simulink model "velo_model"  (R2022a)
settings: Solver=ode1  StartTime=0.0  StopTime=Ts  FixedStep=0.01  RelTol=1e-3
values from neighbouring files (symbols this model uses):
  L = 3    [MultiAgent_initiateSAC.m]    (also in control_velocity.m; initiate.m; initiateHybrid.m; initiateSAC.m)
  ld = 5    [MultiAgent_initiateSAC.m]    (also in control_velocity.m; initiate.m; initiateHybrid.m; initiateSAC.m)
  psi_o = 0    [MultiAgent_initiateSAC.m]    (also in control_velocity.m; initiate.m; initiateHybrid.m = thetaRefs(1)*(pi/180); initiateSAC.m)
  Ts = 100    [MultiAgent_initiateSAC.m]    (also in control_velocity.m; initiate.m; initiateHybrid.m = 50; initiateSAC.m)
  vel = 5    [MultiAgent_initiateSAC.m]    (also in control_velocity.m = 7; initiate.m = 10; initiateHybrid.m; initiateSAC.m)
  X_o = refPose(1,1)+0    [MultiAgent_initiateSAC.m]    (also in control_velocity.m; initiate.m = refPose(1,1)+60; initiateHybrid.m = xRef(1); initiateSAC.m)
  xRef = refPose(:,1)    [MultiAgent_initiateSAC.m]    (also in control_velocity.m; initiate.m; initiateHybrid.m; initiateSAC.m)
  Y_o = -refPose(1,2)+20    [MultiAgent_initiateSAC.m]    (also in control_velocity.m = -refPose(1,2)+0; initiate.m; initiateHybrid.m = yRef(1); initiateSAC.m = -refPose(1,2)+0)
  yRef = -refPose(:,2)    [MultiAgent_initiateSAC.m]    (also in control_velocity.m; initiate.m; initiateHybrid.m; initiateSAC.m)
libraries: vehdynlibviscommon x1, robotalgslib x1, rllib x1, autolibshared x1
settings Model: Creator=berka  LastModifiedBy=berka
settings DebuggingCC: UnconnectedInputMsg=warning  UnconnectedOutputMsg=warning  UnconnectedLineMsg=warning
settings RTWCC: DLArmComputeVersion=19.05

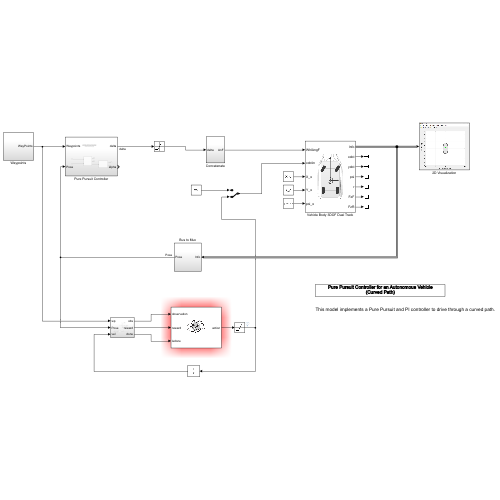
[thumbnail: Simulink's stored preview of the top-level diagram]
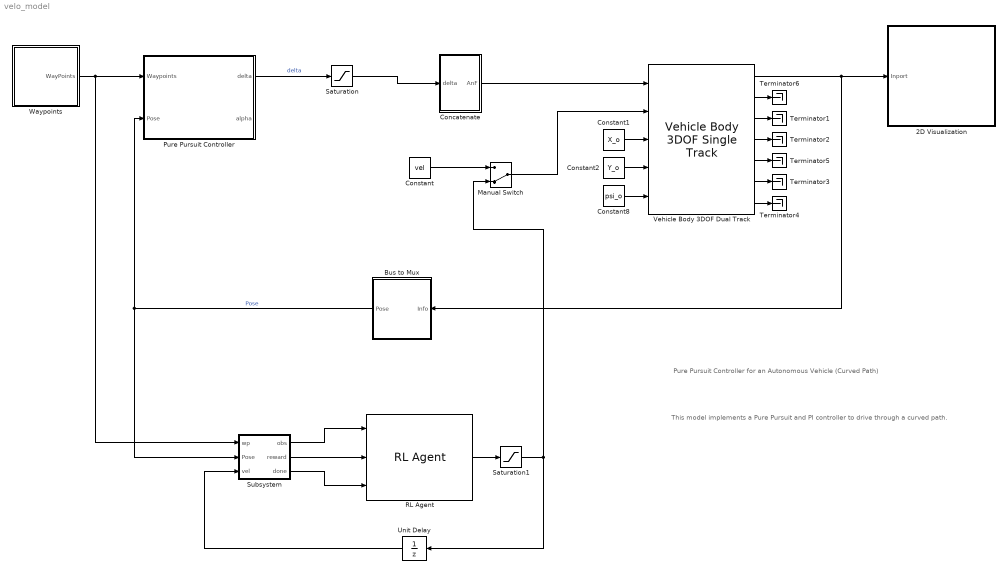
== system velo_model ==
  note: This model implements a Pure Pursuit and PI controller to drive through a curved path.
  note: Pure Pursuit Controller for an Autonomous Vehicle
      | (Curved Path)
  2D Visualization : Subsystem
      mask Display: image("visualization.JPG");
  Bus to Mux : Subsystem
  Concatenate : Subsystem
  Constant : Constant  Value=vel
  Constant1 : Constant  Value=X_o
  Constant2 : Constant  Value=Y_o
  Constant8 : Constant  Value=psi_o
  Manual Switch : ManualSwitch  CurrentSetting=0
  Pure Pursuit Controller : Subsystem
  RL Agent : rllib/RL Agent  Agent=agent  ExternalActionAsInput=off  ProvideLastAction=off  ProvideCumRwd=off  TreatAsDirectFeedthrough=on  UseStrictObservationDataTypes=off
  Saturation : Saturate
  Saturation1 : Saturate  UpperLimit=15  LowerLimit=1
  Subsystem : Subsystem
  Terminator{1..6} (6 alike) : Terminator
  Unit Delay : UnitDelay  SampleTime=-1  HasFrameUpgradeWarning=on
  Vehicle Body 3DOF Dual Track : autolibshared/Vehicle Body 3DOF Single Track  trackMode=Dual  inputMode=External longitudinal velocity  frontSteerMode=on  rearSteerMode=off  windMode=off  muMode=off  extFMode=off  extMMode=off  htchFMode=off  htchMMode=off  extXo=on  extpsio=on  extxdoto=off  extro=off  extYo=on  extTamb=off  extydoto=off  aMode=2  NF=2  NR=2  m=2000  a=1.4  b=1.6  h=0.35  dh=1  hh=0.2  X_o=0  xdot_o=0  CalphaMode=off  sigmaMode=on  d=0  hl=0  w=[1.4,1.4]  Cy_f=12e3  Cy_r=11e3  sigma_f=.1  sigma_r=.1  alpha_f_brk=[-.1 .1]  Cy_f_data=[-9e3 9e3]  alpha_r_brk=[-.1 .1]  Cy_r_data=[-9e3 9e3]  Y_o=0  ydot_o=0  Izz=4000  psi_o=0  r_o=0  Af=2  Cd=.3  Cl=.1  Cpm=.1  beta_w=[0:0.01:0.3]  Cs=[0:0.03:0.9]  Cym=[0:0.01:0.3]  Pabs=101325  Tair=273  g=9.81  mu=1  xdot_tol=.01  Fznom=5000  Fxtire_sat=7e4  Fytire_sat=7e4  longOff=0  latOff=0  vertOff=0  wrapAng=off
      settings: SourceProductBaseCode=PW,DR,MT,VE
  Waypoints : Subsystem
  wires:
  Vehicle Body 3DOF Dual Track/2 -> Terminator6/1
  Constant1/1 -> Vehicle Body 3DOF Dual Track/3
  Vehicle Body 3DOF Dual Track/3 -> Terminator1/1
  Vehicle Body 3DOF Dual Track/1 -> 2D Visualization/1(Inport), Bus to Mux/1(Info)
  Constant8/1 -> Vehicle Body 3DOF Dual Track/5
  Concatenate/1(AnF) -> Vehicle Body 3DOF Dual Track/1
  Vehicle Body 3DOF Dual Track/6 -> Terminator3/1
  Constant2/1 -> Vehicle Body 3DOF Dual Track/4
  Vehicle Body 3DOF Dual Track/7 -> Terminator4/1
  Vehicle Body 3DOF Dual Track/4 -> Terminator2/1
  Vehicle Body 3DOF Dual Track/5 -> Terminator5/1
  Waypoints/1(WayPoints) -> Subsystem/1(wp), Pure Pursuit Controller/1(Waypoints)
  Bus to Mux/1(Pose) -> Subsystem/2(Pose), Pure Pursuit Controller/2(Pose)  "Pose"
  Saturation/1 -> Concatenate/1(delta)
  Pure Pursuit Controller/1(delta) -> Saturation/1  "delta"
  Subsystem/1(obs) -> RL Agent/1
  Subsystem/2(reward) -> RL Agent/2
  Subsystem/3(done) -> RL Agent/3
  RL Agent/1 -> Saturation1/1
  Saturation1/1 -> Unit Delay/1, Manual Switch/2
  Unit Delay/1 -> Subsystem/3(vel)
  Manual Switch/1 -> Vehicle Body 3DOF Dual Track/2
  Constant/1 -> Manual Switch/1

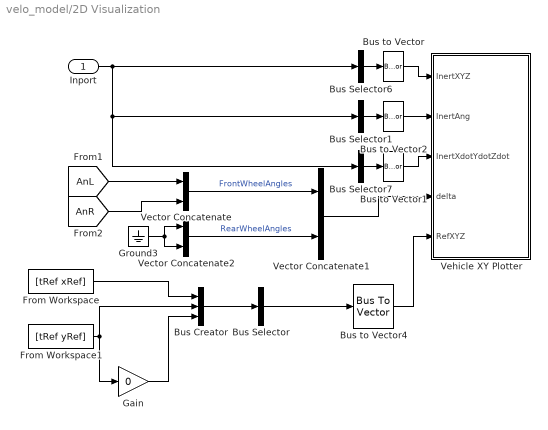
== system velo_model/2D Visualization ==
  Inport : Inport
  Bus Creator : BusCreator  Inputs=3
  Bus Selector : BusSelector  OutputSignals=signal1,signal2,signal3  OutputAsBus=on
  Bus Selector1 : BusSelector  OutputSignals=InertFrm.Cg.Ang.phi,InertFrm.Cg.Ang.theta,InertFrm.Cg.Ang.psi  OutputAsBus=on
  Bus Selector6 : BusSelector  OutputSignals=InertFrm.Geom.Disp.X,InertFrm.Geom.Disp.Y,InertFrm.Geom.Disp.Z  OutputAsBus=on
  Bus Selector7 : BusSelector  OutputSignals=InertFrm.Geom.Vel.Xdot,InertFrm.Geom.Vel.Ydot,InertFrm.Geom.Vel.Zdot  OutputAsBus=on
  Bus to Vector{,1..2,4} (4 alike) : BusToVector
  From Workspace : FromWorkspace  VariableName=[tRef xRef]
  From Workspace1 : FromWorkspace  VariableName=[tRef yRef]
  Gain : Gain  Gain=0
  Ground3 : Ground
  Vector Concatenate : Concatenate
  Vector Concatenate1 : Concatenate
  Vector Concatenate2 : Concatenate
  Vehicle XY Plotter : Subsystem  mask(Vehicle XY Plotter){a=2, b=2, w=2, figBorder=10, bufferSize=1024, extRef=on, pltDT=.2}
      mask prompts: a "Distance to front axle from CG, a [m]:"; b "Distance to rear axle from CG, b [m]:"; w "Track width, w [m]:"; figBorder "Distance to figure borders, figBorder [m]:"; bufferSize "Path buffer sampe size, bufferSize []:"; extRef "Plot path reference, extRef"; pltDT "Plot update rate, pltDT [s]:"
      mask help:
      | This block will display a MATLAB figure which indicates the vehicle path, current position and heading velocity.
      | An optional path reference is also provided.
      mask init:
      | if autoblkschecksimstopped(gcb)
      |     PortName = 'RefXYZ';
      |     InportOption  = {'built-in/Ground', [PortName, ' Ground'];...
      |         'built-in/Inport',PortName };
      |     if ~strcmp(get_param(gcb,'extRef'),'on')
      |         NewBlkHdl = autoblksreplaceblock(gcb, InportOption, 1);
      |         set_param(NewBlkHdl, 'ShowName', 'off');
      |     else
      |         autoblksreplaceblock(gcb, InportOption, 2);
      |     end
      | end
      mask TypeOptions a: Vehicle XY Plotter/a
      mask TypeOptions b: Vehicle XY Plotter/b
      mask TypeOptions w: Vehicle XY Plotter/w
      mask TypeOptions figBorder: Vehicle XY Plotter/figBorder
      mask TypeOptions bufferSize: Vehicle XY Plotter/bufferSize
  wires:
  Vector Concatenate1/1 -> Vehicle XY Plotter/4(delta)
  Ground3/1 -> Vector Concatenate2/1, Vector Concatenate2/2
  Bus Selector6/1 -> Bus to Vector/1
  Vector Concatenate/1 -> Vector Concatenate1/1  "FrontWheelAngles"
  [AnL] -> Vector Concatenate/1
  Vector Concatenate2/1 -> Vector Concatenate1/2  "RearWheelAngles"
  Bus Selector7/1 -> Bus to Vector1/1
  Bus to Vector1/1 -> Vehicle XY Plotter/3(InertXdotYdotZdot)
  Bus to Vector/1 -> Vehicle XY Plotter/1(InertXYZ)
  Bus to Vector2/1 -> Vehicle XY Plotter/2(InertAng)
  Bus Selector1/1 -> Bus to Vector2/1
  [AnR] -> Vector Concatenate/2
  Inport/1 -> Bus Selector7/1, Bus Selector1/1, Bus Selector6/1
  Bus to Vector4/1 -> Vehicle XY Plotter/5(RefXYZ)
  Bus Selector/1 -> Bus to Vector4/1
  From Workspace1/1 -> Gain/1, Bus Creator/2
  Gain/1 -> Bus Creator/3
  From Workspace/1 -> Bus Creator/1
  Bus Creator/1 -> Bus Selector/1

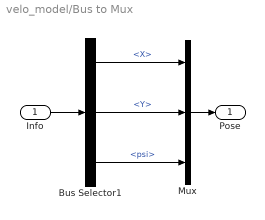
== system velo_model/Bus to Mux ==
  Info : Inport
  Bus Selector1 : BusSelector  OutputSignals=InertFrm.Cg.Disp.X,InertFrm.Cg.Disp.Y,InertFrm.Cg.Ang.psi
  Mux : Mux  Inputs=3
  Pose : Outport
  wires:
  Bus Selector1/3 -> Mux/3  "<psi>"
  Bus Selector1/1 -> Mux/1  "<X>"
  Mux/1 -> Pose/1
  Bus Selector1/2 -> Mux/2  "<Y>"
  Info/1 -> Bus Selector1/1

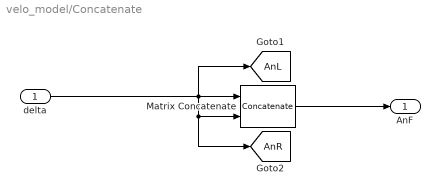
== system velo_model/Concatenate ==
  delta : Inport
  Matrix Concatenate : Concatenate
  AnF : Outport  VectorParamsAs1DForOutWhenUnconnected=off
  tag scope: AnL=global, AnR=global
  wires:
  Matrix Concatenate/1 -> AnF/1
  delta/1 -> [AnL], [AnR], Matrix Concatenate/2, Matrix Concatenate/1

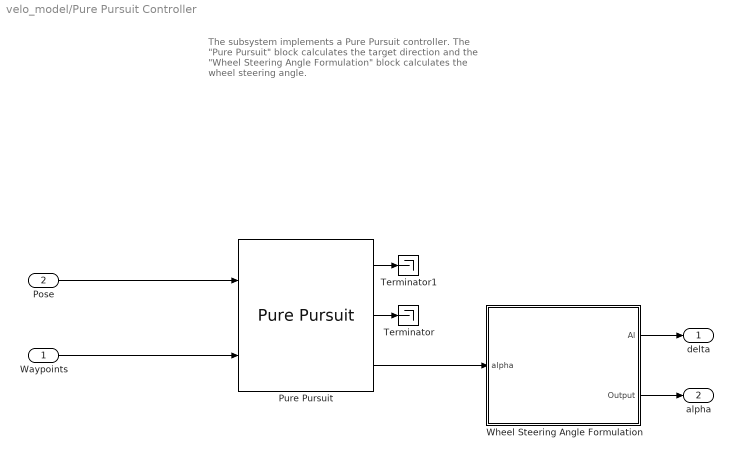
== system velo_model/Pure Pursuit Controller ==
  note: The subsystem implements a Pure Pursuit controller. The "Pure Pursuit" block calculates the target direction and the "Wheel Steering Angle Formulation" block calculates the wheel steering angle.
  Waypoints : Inport
  Pose : Inport  Port=2
  Pure Pursuit : robotalgslib/Pure Pursuit  DesiredLinearVelocity=vel  MaxAngularVelocity=1.0  LookaheadDistance=2.2754  TargetDirPort=on  SimulateUsing=Code generation
  Terminator : Terminator
  Terminator1 : Terminator
  Wheel Steering Angle Formulation : Subsystem  mask{L=L, ld=ld}
      mask prompts: L "Bicycle length"; ld "Lookahead distance"
      mask TypeOptions L: Bicycle length/Value
      mask TypeOptions ld: Lookahead distance/Value
      mask Display:
      | image("GeometryMask.png")
      | port_label('input', 1, 'alpha')
      | port_label('output', 1, 'delta')
  delta : Outport
  alpha : Outport  Port=2
  wires:
  Pure Pursuit/3 -> Wheel Steering Angle Formulation/1(alpha)
  Waypoints/1 -> Pure Pursuit/2
  Pose/1 -> Pure Pursuit/1
  Pure Pursuit/1 -> Terminator1/1
  Pure Pursuit/2 -> Terminator/1
  Wheel Steering Angle Formulation/1(Al) -> delta/1
  Wheel Steering Angle Formulation/2(Output) -> alpha/1

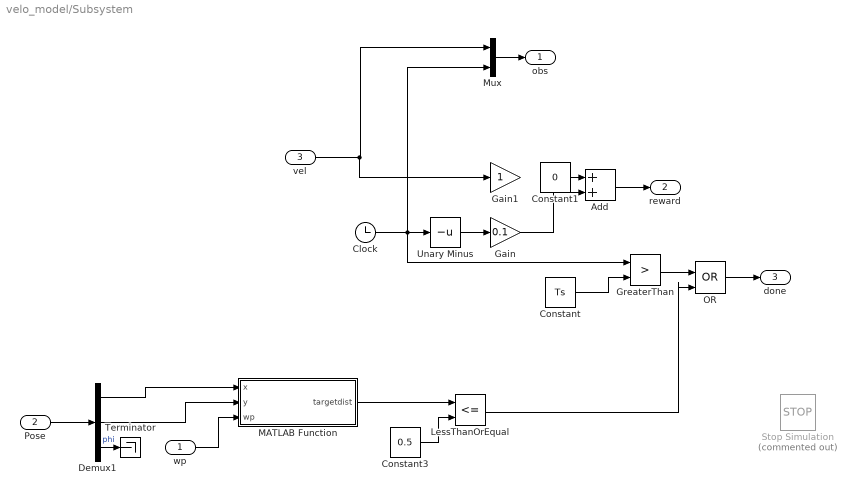
== system velo_model/Subsystem ==
  wp : Inport
  Pose : Inport  Port=2
  vel : Inport  Port=3
  Add : Sum
  Clock : Clock
  Constant : Constant  Value=Ts
  Constant1 : Constant  Value=0
  Constant3 : Constant  Value=0.5
  Demux1 : Demux  Outputs=3
  Gain : Gain  Gain=0.1
  Gain1 : Gain
  GreaterThan : RelationalOperator  Operator=>  OutDataTypeStr=boolean  RndMeth=Simplest  InputSameDT=off
  LessThanOrEqual : RelationalOperator  Operator=<=  OutDataTypeStr=boolean  RndMeth=Simplest  InputSameDT=off
  MATLAB Function : MATLAB Function  TreatAsAtomicUnit=on
  Mux : Mux  Inputs=2
  OR : Logic  Operator=OR  IconShape=distinctive  AllPortsSameDT=off  OutDataTypeStr=boolean
  Stop Simulation : Stop  Commented=on
  Terminator : Terminator
  Unary Minus : UnaryMinus
  obs : Outport
  reward : Outport  Port=2
  done : Outport  Port=3
  wires:
  Demux1/3 -> Terminator/1  "phi"
  Constant3/1 -> LessThanOrEqual/2
  Clock/1 -> GreaterThan/1, Mux/2, Unary Minus/1
  Pose/1 -> Demux1/1
  Unary Minus/1 -> Gain/1
  Demux1/1 -> MATLAB Function/1(x)
  MATLAB Function/1(targetdist) -> LessThanOrEqual/1
  Demux1/2 -> MATLAB Function/2(y)
  wp/1 -> MATLAB Function/3(wp)
  vel/1 -> Gain1/1, Mux/1
  Mux/1 -> obs/1
  Add/1 -> reward/1
  Gain/1 -> Add/2
  Constant/1 -> GreaterThan/2
  GreaterThan/1 -> OR/1
  LessThanOrEqual/1 -> OR/2
  OR/1 -> done/1
  Constant1/1 -> Add/1

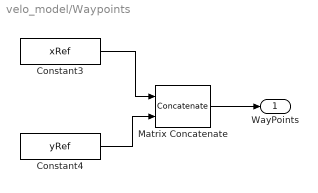
== system velo_model/Waypoints ==
  Constant3 : Constant  Value=xRef  SampleTime=0.1
  Constant4 : Constant  Value=yRef  SampleTime=0.1
  Matrix Concatenate : Concatenate  Mode=Multidimensional array  ConcatenateDimension=2
  WayPoints : Outport
  wires:
  Constant4/1 -> Matrix Concatenate/2
  Matrix Concatenate/1 -> WayPoints/1
  Constant3/1 -> Matrix Concatenate/1

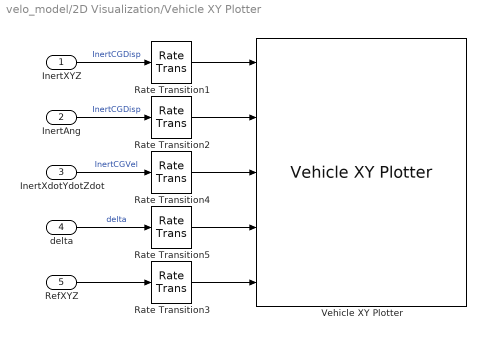
== system velo_model/2D Visualization/Vehicle XY Plotter ==
  InertXYZ : Inport
  InertAng : Inport  Port=2
  InertXdotYdotZdot : Inport  Port=3
  delta : Inport  Port=4
  RefXYZ : Inport  Port=5
  Rate Transition{1..5} (5 alike) : RateTransition  Deterministic=off  OutPortSampleTime=pltDT
  Vehicle XY Plotter : vehdynlibviscommon/Vehicle XY Plotter  w=w  a=a  b=b  figBorder=figBorder  bufferSize=bufferSize  extStats=off  extTireF=off
      settings: SourceProductBaseCode=VE
  wires:
  Rate Transition5/1 -> Vehicle XY Plotter/4
  Rate Transition4/1 -> Vehicle XY Plotter/3
  Rate Transition2/1 -> Vehicle XY Plotter/2
  Rate Transition1/1 -> Vehicle XY Plotter/1
  Rate Transition3/1 -> Vehicle XY Plotter/5
  delta/1 -> Rate Transition5/1  "delta"
  InertXYZ/1 -> Rate Transition1/1  "InertCGDisp"
  InertXdotYdotZdot/1 -> Rate Transition4/1  "InertCGVel"
  InertAng/1 -> Rate Transition2/1  "InertCGDisp"
  RefXYZ/1 -> Rate Transition3/1

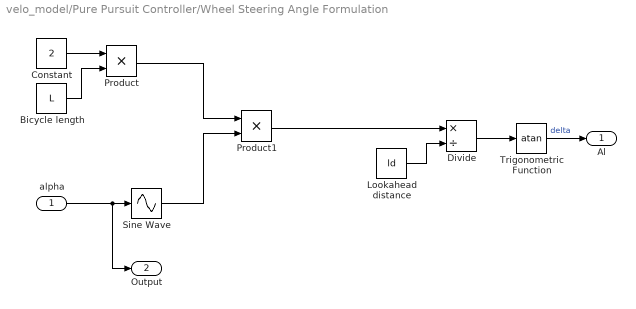
== system velo_model/Pure Pursuit Controller/Wheel Steering Angle Formulation ==
  alpha : Inport
  Bicycle length : Constant  Value=L
  Constant : Constant  Value=2
  Divide : Product  Inputs=*/
  Lookahead distance : Constant  Value=ld
  Product : Product
  Product1 : Product
  Sine Wave : Sin  TimeSource=Use external signal  SampleTime=0
  Trigonometric Function : Trigonometry  Operator=atan
  Al : Outport
  Output : Outport  Port=2
  wires:
  Sine Wave/1 -> Product1/2
  Bicycle length/1 -> Product/2
  Constant/1 -> Product/1
  Product1/1 -> Divide/1
  Product/1 -> Product1/1
  Divide/1 -> Trigonometric Function/1
  Trigonometric Function/1 -> Al/1  "delta"
  alpha/1 -> Output/1, Sine Wave/1
  Lookahead distance/1 -> Divide/2

== matlab function velo_model/Subsystem/MATLAB Function ==
  data: x input; targetdist output; y input; wp input
function targetdist  = fcn(x,y,wp)

x_last = wp(end,1);
y_last = wp(end,2);
targetdist = sqrt((x_last-x)^2 + (y_last-y)^2);

end
